simulink model "minJerkTrajMDL"  (Simulink 7.9)
settings: Solver=ode3  StartTime=0.0  StopTime=inf  RelTol=1e-3
settings Model: Creator=jorhabib  LastModifiedBy=daniele

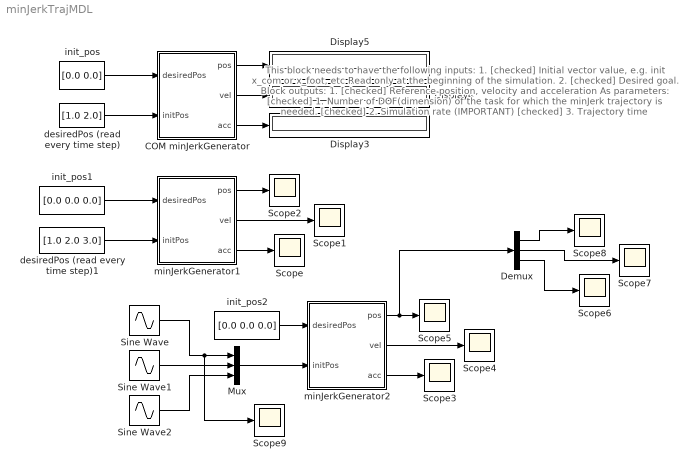
== system minJerkTrajMDL ==
  note: This block needs to have the following inputs:
      | 1. [checked] Initial vector value, e.g. init x_com or x_foot, etc Read only
      |                     at the beginning of the simulation.
      | 2. [checked] Desired goal.
      |
      | Block outputs:
      | 1. [checked] Reference position, velocity and acceleration
      |
      | As parameters:
      | [checked] 1. Number of DOF(dimension) of the task for which the minJerk
      | trajectory is needed.
      | [checked] 2. Simulation rate (IMPORTANT)
      | [checked] 3. Trajectory time
  COM minJerkGenerator : Subsystem
  Demux : Demux  Outputs=3
  Display3 : Display
  Display4 : Display
  Display5 : Display
  Mux : Mux  Inputs=3
  Scope{,1..9} (10 alike) : Scope
      Scope settings: YMin=-0.275  YMax=-0.075
      Scope1 settings: YMin=0.15  YMax=0.7
      Scope2 settings: YMin=0.9  YMax=3  SaveName=ScopeData2
      Scope3 settings: YMin=-0.275  YMax=-0.075  SaveName=ScopeData3
      Scope4 settings: YMin=0.15  YMax=0.7  SaveName=ScopeData4
      Scope5 settings: YMin=-1  YMax=1  SaveName=ScopeData5
      Scope6 settings: YMin=-0.0175  YMax=0.0175  SaveName=ScopeData6
      Scope7 settings: YMin=-0.0175  YMax=0.0175  SaveName=ScopeData7
      Scope8 settings: YMin=-0  YMax=0.09  SaveName=ScopeData8
      Scope9 settings: YMin=-1  YMax=1  SaveName=ScopeData9
  Sine Wave : Sin  Frequency=2*pi/(4*10e-3)
  Sine Wave1 : Sin
  Sine Wave2 : Sin  Frequency=10000
  desiredPos (read every time step) : Constant  Value=[1.0 2.0]  OutDataTypeStr=double
  desiredPos (read every time step)1 : Constant  Value=[1.0 2.0 3.0]  OutDataTypeStr=double
  init_pos : Constant  Value=[0.0 0.0]  OutDataTypeStr=double
  init_pos1 : Constant  Value=[0.0 0.0 0.0]  OutDataTypeStr=double
  init_pos2 : Constant  Value=[0.0 0.0 0.0]  OutDataTypeStr=double
  minJerkGenerator1 : Subsystem
  minJerkGenerator2 : Subsystem
  wires:
  init_pos/1 -> COM minJerkGenerator/1(desiredPos)
  desiredPos (read every time step)/1 -> COM minJerkGenerator/2(initPos)
  COM minJerkGenerator/1(pos) -> Display5/1
  COM minJerkGenerator/2(vel) -> Display4/1
  COM minJerkGenerator/3(acc) -> Display3/1
  init_pos1/1 -> minJerkGenerator1/1(desiredPos)
  desiredPos (read every time step)1/1 -> minJerkGenerator1/2(initPos)
  minJerkGenerator1/2(vel) -> Scope1/1
  minJerkGenerator1/3(acc) -> Scope/1
  minJerkGenerator1/1(pos) -> Scope2/1
  Sine Wave/1 -> Mux/1, Scope9/1
  Sine Wave1/1 -> Mux/2
  Sine Wave2/1 -> Mux/3
  minJerkGenerator2/2(vel) -> Scope4/1
  minJerkGenerator2/3(acc) -> Scope3/1
  minJerkGenerator2/1(pos) -> Scope5/1, Demux/1
  init_pos2/1 -> minJerkGenerator2/1(desiredPos)
  Mux/1 -> minJerkGenerator2/2(initPos)
  Demux/1 -> Scope8/1
  Demux/2 -> Scope7/1
  Demux/3 -> Scope6/1

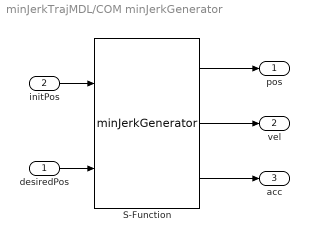
== system minJerkTrajMDL/COM minJerkGenerator ==
  desiredPos : Inport
  initPos : Inport  Port=2
  S-Function : S-Function  FunctionName=minJerkGenerator  Parameters=dim, rate, tt  EnableBusSupport=off  mask{dim=2, rate=10, tt=4}
      mask prompts: dim "Trajectory dimension (int)"; rate "Simulation rate (int) [ms]"; tt "Trajectory time [s]"
  pos : Outport
  vel : Outport  Port=2
  acc : Outport  Port=3
  wires:
  S-Function/2 -> vel/1
  S-Function/1 -> pos/1
  S-Function/3 -> acc/1
  initPos/1 -> S-Function/1
  desiredPos/1 -> S-Function/2

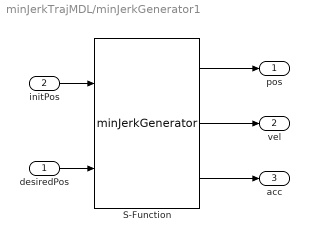
== system minJerkTrajMDL/minJerkGenerator1 ==
  desiredPos : Inport
  initPos : Inport  Port=2
  S-Function : S-Function  FunctionName=minJerkGenerator  Parameters=dim, rate, tt  EnableBusSupport=off  mask{dim=3, rate=10, tt=1}
      mask prompts: dim "Trajectory dimension (int)"; rate "Simulation rate (int) [ms]"; tt "Trajectory time [s]"
  pos : Outport
  vel : Outport  Port=2
  acc : Outport  Port=3
  wires:
  desiredPos/1 -> S-Function/2
  initPos/1 -> S-Function/1
  S-Function/3 -> acc/1
  S-Function/1 -> pos/1
  S-Function/2 -> vel/1

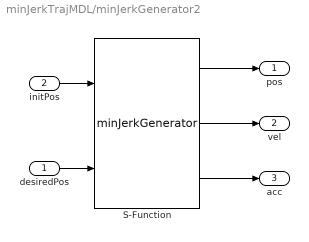
== system minJerkTrajMDL/minJerkGenerator2 ==
  desiredPos : Inport
  initPos : Inport  Port=2
  S-Function : S-Function  FunctionName=minJerkGenerator  Parameters=dim, rate, tt  EnableBusSupport=off  mask{dim=3, rate=10, tt=0.05}
      mask prompts: dim "Trajectory dimension (int)"; rate "Simulation rate (int) [ms]"; tt "Trajectory time [s]"
  pos : Outport
  vel : Outport  Port=2
  acc : Outport  Port=3
  wires:
  S-Function/2 -> vel/1
  S-Function/1 -> pos/1
  S-Function/3 -> acc/1
  initPos/1 -> S-Function/1
  desiredPos/1 -> S-Function/2
